simulink model "dvbs2_stream"  (R2024b)
settings: Solver=FixedStepDiscrete  StartTime=0.0  StopTime=18000/Fs  RelTol=1e-3
PreLoadFcn:
  | Rs = 125e3;
  | Fs = 8*Rs;
  | nsamp = 4096;
  | t = (0:nsamp)/Fs;
  | y = randi(2^8-1,1,2048);
  | ly = length(y);
InitFcn:
  | Rs = 125e3;
  | Fs = 8*Rs;
  | nsamp = 4096;
  | t = (0:nsamp)/Fs;
  | y = randi(2^8-1,1,2048);
  | ly = length(y);
libraries: hdlsllib x132, simulink x41, dspsigops x7, commseqgen3 x5, whdlutilities x5, commhdlcrc x2, dsphdlfiltering2 x1, whdlmod x1, sdrzblksprivate x1
(part 4 of 6)

== system dvbs2_stream/HDL_DUT/Tx/DVB-S2 Tx/PL Frame Generator/RAM FIFO/PL Header FIFO ==
  dataIn : Inport
  validIn : Inport  Port=2
  nextFrameReady : Inport  Port=3
  90x : MATLAB Function  TreatAsAtomicUnit=on
  Delay{1..3,9} (4 alike) : Delay  DelayLength=1
  HDL Counter2 : hdlsllib/Sources/HDL Counter  CountType=Count limited  CountInit=0  CountStep=1  CountMax=2^9 - 1  CountFromType=Initial value  CountFrom=0  CountResetPort=off  CountLoadPort=off  CountEnbPort=on  CountDirPort=off  CountHitOutputPort=off  CountDataType=Unsigned  CountWordLen=nextpow2(450)  CountFracLen=0  CountSampTime=1
  HDL Counter3 : hdlsllib/Sources/HDL Counter  CountType=Count limited  CountInit=0  CountStep=1  CountMax=2^9 - 1  CountFromType=Initial value  CountFrom=0  CountResetPort=off  CountLoadPort=off  CountEnbPort=on  CountDirPort=off  CountHitOutputPort=off  CountDataType=Unsigned  CountWordLen=nextpow2(450)  CountFracLen=0  CountSampTime=1
  No HDL : Subsystem
  Simple Dual Port RAM : hdlsllib/HDL RAMs/Simple Dual Port RAM  ram_size=nextpow2(450)
  dataOut : Outport
  startOut : Outport  Port=2
  endOut : Outport  Port=3
  validOut : Outport  Port=4
  endOut1 : Outport  Port=5
  wires:
  90x/4(endOutm1) -> Delay3/1
  Delay3/1 -> endOut1/1
  Delay2/1 -> endOut/1
  Delay1/1 -> startOut/1
  Delay9/1 -> validOut/1
  Simple Dual Port RAM/1 -> dataOut/1
  nextFrameReady/1 -> 90x/1(trigger)
  90x/3(endOut) -> Delay2/1
  90x/2(startOut) -> Delay1/1
  90x/1(validOut) -> Delay9/1, No HDL/2(rd), HDL Counter3/1
  HDL Counter2/1 -> Simple Dual Port RAM/2
  dataIn/1 -> Simple Dual Port RAM/1
  HDL Counter3/1 -> Simple Dual Port RAM/4
  validIn/1 -> No HDL/1(wr), HDL Counter2/1, Simple Dual Port RAM/3

== system dvbs2_stream/HDL_DUT/Tx/DVB-S2 Tx/PL Frame Generator/RAM FIFO/Pilot Generator ==
  trigger : Inport
  Pilot Block Length Valid Generator : MATLAB Function  TreatAsAtomicUnit=on
  Pilot or Unmodulated Carrier : Constant  Value=fi(exp(1i*pi/4),1,18,16)  SampleTime=1/Rsym
  dataOut : Outport
  endOut : Outport  Port=2
  validOut : Outport  Port=3
  endOut1 : Outport  Port=4
  wires:
  Pilot Block Length Valid Generator/2(endOutm1) -> endOut1/1
  Pilot Block Length Valid Generator/3(validOut) -> validOut/1
  Pilot Block Length Valid Generator/1(endOut) -> endOut/1
  Pilot or Unmodulated Carrier/1 -> dataOut/1
  trigger/1 -> Pilot Block Length Valid Generator/1(trigger)

== system dvbs2_stream/HDL_DUT/Tx/DVB-S2 Tx/BB Frame Generator/BB Header and Data CRC Generator/Data Field Generator/Continuous Streams ==
  dataIn : Inport
  validIn : Inport  Port=2
  frameEnd : Inport  Port=3
  frameStart : Inport  Port=4
  Delay{,1..3} (4 alike) : Delay  DelayLength=8+1+10
  dataOut : Outport
  validOut : Outport  Port=2
  frameEndOut : Outport  Port=3
  frameStartOut : Outport  Port=4
  wires:
  validIn/1 -> Delay1/1
  frameEnd/1 -> Delay2/1
  Delay2/1 -> frameEndOut/1
  Delay3/1 -> frameStartOut/1
  frameStart/1 -> Delay3/1
  Delay1/1 -> validOut/1
  dataIn/1 -> Delay/1
  Delay/1 -> dataOut/1

== system dvbs2_stream/HDL_DUT/Tx/DVB-S2 Tx/BB Frame Generator/BB Header and Data CRC Generator/Data Field Generator/Packetized Streams ==
  dataIn : Inport
  startIn : Inport  Port=2
  endIn : Inport  Port=3
  validIn : Inport  Port=4
  frameEnd : Inport  Port=5
  frameStart : Inport  Port=6
  Delay : Delay  DelayLength=1
  Delay1 : Delay  DelayLength=1
  Delay2 : Delay  DelayLength=8
  Delay3 : Delay  DelayLength=10
  Delay4 : Delay  DelayLength=10
  Discard SYNC : MATLAB Function  TreatAsAtomicUnit=on
  MATLAB Function : MATLAB Function  TreatAsAtomicUnit=on
  Terminator : Terminator
  Terminator1 : Terminator
  User Packet CRC Generator : commhdlcrc/General CRC Generator HDL Optimized  Polynomial=[1 1 1 0 1 0 1 0 1]  InitialState=0  DirectMethod=off  ReflectInput=off  ReflectCRCChecksum=off  FinalXORValue=0  SimulateUsing=Code generation
  pktBits : Outport
  pktValid : Outport  Port=2
  frameEndOut : Outport  Port=3
  frameStartOut : Outport  Port=4
  wires:
  Delay4/1 -> MATLAB Function/2(frameEndIn)
  User Packet CRC Generator/4 -> pktValid/1
  Delay3/1 -> frameStartOut/1
  endIn/1 -> Discard SYNC/3(endIn)
  startIn/1 -> Discard SYNC/2(startIn)
  frameEnd/1 -> Delay/1
  frameStart/1 -> Delay2/1
  User Packet CRC Generator/1 -> pktBits/1
  Delay1/1 -> Delay3/1
  Discard SYNC/2(startOut) -> User Packet CRC Generator/2
  Discard SYNC/3(endOut) -> User Packet CRC Generator/3
  User Packet CRC Generator/2 -> Terminator/1
  User Packet CRC Generator/3 -> MATLAB Function/1(pktEndIn), Terminator1/1
  Discard SYNC/4(validOut) -> User Packet CRC Generator/4
  dataIn/1 -> Discard SYNC/1(dataIn)
  validIn/1 -> Discard SYNC/4(validIn)
  Delay/1 -> Delay4/1
  Delay2/1 -> Delay1/1
  MATLAB Function/1(frameEndOut) -> frameEndOut/1
  Discard SYNC/1(dataOut) -> User Packet CRC Generator/1

== system dvbs2_stream/HDL_DUT/Tx/DVB-S2 Tx/BB Frame Generator/BB Header and Data CRC Generator/No HDL/No HDL ==
  rdy : Inport
  vld : Inport  Port=2
  Assertion : Assertion
  Logical Operator : Logic  AllPortsSameDT=off  OutDataTypeStr=boolean
  Logical Operator1 : Logic  Operator=NOT  AllPortsSameDT=off  OutDataTypeStr=boolean
  Logical Operator2 : Logic  Operator=NOT  AllPortsSameDT=off  OutDataTypeStr=boolean
  wires:
  Logical Operator2/1 -> Assertion/1
  rdy/1 -> Logical Operator1/1
  Logical Operator/1 -> Logical Operator2/1
  vld/1 -> Logical Operator/2
  Logical Operator1/1 -> Logical Operator/1

== system dvbs2_stream/HDL_DUT/Tx/DVB-S2 Tx/BB Frame Generator/Data Store FIFO/No HDL/No HDL ==
  wr : Inport
  full : Inport  Port=2
  ncount : Inport  Port=3
  empty : Inport  Port=4
  rd : Inport  Port=5
  Assertion : Assertion  AssertionFailFcn=warning('push on to a full RAM');  StopWhenAssertionFail=off
  Assertion1 : Assertion  AssertionFailFcn=warning('pop from an empty RAM');  StopWhenAssertionFail=off
  Assertion2 : Assertion  AssertionFailFcn='count exceeded 80'
  Compare To Constant : simulink/Logic and Bit Operations/Compare To Constant  relop=<=  const=80  OutDataTypeStr=boolean
  Display : Display
  Logical Operator : Logic  Operator=NAND  AllPortsSameDT=off  OutDataTypeStr=boolean
  Logical Operator1 : Logic  Operator=NAND  AllPortsSameDT=off  OutDataTypeStr=boolean
  wires:
  Logical Operator1/1 -> Assertion1/1
  wr/1 -> Logical Operator/1
  full/1 -> Logical Operator/2
  ncount/1 -> Compare To Constant/1, Display/1
  empty/1 -> Logical Operator1/1
  Logical Operator/1 -> Assertion/1
  rd/1 -> Logical Operator1/2
  Compare To Constant/1 -> Assertion2/1

== system dvbs2_stream/HDL_DUT/Tx/DVB-S2 Tx/FEC Encoder/DVB-S2 BCH Encoder/Parity Generation/Store and Retrieve Parity ==
  iwr_data : Inport  Partition=on  PartitionDimension=1  PartitionWidth=1  PartitionOffset=0
  iwr_addr : Inport  Port=2
  iwr_enb : Inport  Port=3  Partition=on  PartitionDimension=1  PartitionWidth=1  PartitionOffset=0
  ird_addr : Inport  Port=4
  For Each : ForEach  DisableCoverage=on
  parity RAM : hdlsllib/HDL RAMs/Simple Dual Port RAM  ram_size=3
  ird_data : Outport  ConcatenationDimension=1
  wires:
  ird_addr/1 -> parity RAM/4
  iwr_data/1 -> parity RAM/1
  iwr_addr/1 -> parity RAM/2
  iwr_enb/1 -> parity RAM/3
  parity RAM/1 -> ird_data/1

== system dvbs2_stream/HDL_DUT/Tx/DVB-S2 Tx/Interleaver/DVB-S2 HDL Interleaver/RAM/Single RAM Using Two RAMs ==
  wr_din : Inport
  wr_addr : Inport  Port=2
  wr_en : Inport  Port=3
  rd_addr : Inport  Port=4
  Delay : Delay  DelayLength=1
  Extract Bits : simulink/Logic and Bit Operations/Extract Bits  bitsToExtract=Range of bits  numBits=8  bitIdxRange=[0 15]  outScalingMode=Treat bit field as an integer
  Extract Bits1 : simulink/Logic and Bit Operations/Extract Bits  bitsToExtract=Range of bits  numBits=8  bitIdxRange=16  outScalingMode=Treat bit field as an integer
  Extract Bits2 : simulink/Logic and Bit Operations/Extract Bits  bitsToExtract=Range of bits  numBits=8  bitIdxRange=[0 15]  outScalingMode=Treat bit field as an integer
  Extract Bits3 : simulink/Logic and Bit Operations/Extract Bits  bitsToExtract=Range of bits  numBits=8  bitIdxRange=16  outScalingMode=Treat bit field as an integer
  Logical Operator1 : Logic  Operator=NOT  AllPortsSameDT=off  OutDataTypeStr=boolean
  Logical Operator2 : Logic  AllPortsSameDT=off  OutDataTypeStr=boolean
  Logical Operator3 : Logic  AllPortsSameDT=off  OutDataTypeStr=boolean
  Multiport Switch : MultiPortSwitch  DataPortOrder=Zero-based contiguous  Inputs=2  zeroidx=on  SaturateOnIntegerOverflow=off  InputSameDT=off
  Simple Dual Port RAM : hdlsllib/HDL RAMs/Simple Dual Port RAM  ram_size=nextpow2(ConfigRx.RAMCapacity/2)
  Simple Dual Port RAM1 : hdlsllib/HDL RAMs/Simple Dual Port RAM  ram_size=nextpow2(ConfigRx.RAMCapacity/2)
  rd_dout : Outport
  wires:
  Delay/1 -> Multiport Switch/1
  Multiport Switch/1 -> rd_dout/1
  Simple Dual Port RAM1/1 -> Multiport Switch/3
  Extract Bits3/1 -> Delay/1
  Extract Bits2/1 -> Simple Dual Port RAM1/4, Simple Dual Port RAM/4
  Logical Operator2/1 -> Simple Dual Port RAM1/3
  Logical Operator3/1 -> Simple Dual Port RAM/3
  Logical Operator1/1 -> Logical Operator3/1
  Extract Bits1/1 -> Logical Operator2/1, Logical Operator1/1
  Extract Bits/1 -> Simple Dual Port RAM1/2, Simple Dual Port RAM/2
  Simple Dual Port RAM/1 -> Multiport Switch/2
  wr_din/1 -> Simple Dual Port RAM/1, Simple Dual Port RAM1/1
  rd_addr/1 -> Extract Bits3/1, Extract Bits2/1
  wr_en/1 -> Logical Operator2/2, Logical Operator3/2
  wr_addr/1 -> Extract Bits1/1, Extract Bits/1

== system dvbs2_stream/HDL_DUT/Tx/DVB-S2 Tx/Interleaver/DVB-S2 HDL Interleaver/RAM/Wrap Address ==
  u : Inport
  Add : Sum  Inputs=+-  OutDataTypeStr=Inherit: Same as first input
  Compare To Constant : simulink/Logic and Bit Operations/Compare To Constant  relop=>=  const=ConfigRx.RAMCapacity  OutDataTypeStr=boolean
  Constant : Constant  Value=ConfigRx.RAMCapacity  OutDataTypeStr=Inherit: Inherit via back propagation  SampleTime=Tsamp
  Constant1 : Constant  Value=0  OutDataTypeStr=Inherit: Inherit via back propagation  SampleTime=Tsamp
  Data Type Duplicate : DataTypeDuplicate
  Data Type Duplicate1 : DataTypeDuplicate
  Data Type Conversion : DataTypeConversion  OutDataTypeStr=fixdt(0,nextpow2(ConfigRx.RAMCapacity),0)  SaturateOnIntegerOverflow=off  RndMeth=Floor
  Switch : Switch  Criteria=u2 ~= 0  SaturateOnIntegerOverflow=off  InputSameDT=off
  Switch1 : Switch  Criteria=u2 ~= 0  SaturateOnIntegerOverflow=off  InputSameDT=off
  y : Outport
  wires:
  u/1 -> Switch/3, Data Type Duplicate/1, Add/1, Compare To Constant/1
  Switch/1 -> Data Type Conversion/1
  Compare To Constant/1 -> Switch1/2, Switch/2
  Add/1 -> Switch/1
  Constant/1 -> Switch1/1, Data Type Duplicate1/1, Data Type Duplicate/2
  Data Type Conversion/1 -> y/1
  Switch1/1 -> Add/2
  Constant1/1 -> Data Type Duplicate1/2, Switch1/3

== system dvbs2_stream/HDL_DUT/Tx/DVB-S2 Tx/Interleaver/DVB-S2 HDL Interleaver/RAM Address Generator/Generate and Add Read Base Address ==
  readAddrIn : Inport
  readValidIn : Inport  Port=2
  startIn : Inport  Port=3
  endIn : Inport  Port=4
  Add : Sum  Inputs=|++
  Delay{,1,3..4,18} (5 alike) : Delay  DelayLength=1
  Delay{5..9,11,13..16,19..20} (12 alike) : Delay
  Gain : Gain  Gain=ConfigRx.ShortFrameLen  ParamDataTypeStr=fixdt(0,nextpow2(16200),0)
  HDL Counter : hdlsllib/Sources/HDL Counter  CountType=Count limited  CountInit=0  CountStep=1  CountMax=(ConfigRx.RAMCapacity/ConfigRx.ShortFrameLen) - 1  CountFromType=Initial value  CountFrom=0  CountResetPort=off  CountLoadPort=off  CountEnbPort=on  CountDirPort=off  CountHitOutputPort=off  CountDataType=Unsigned  CountWordLen=nextpow2((ConfigRx.RAMCapacity/ConfigRx.ShortFrameLen) - 1)  CountFracLen=0  CountSampTime=1
  Indicate End of Every ShortFrame Length Samples : Subsystem
  Logical Operator : Logic  AllPortsSameDT=off  OutDataTypeStr=boolean
  No HDL Read Address Debug Scope : Subsystem
      settings: PortSchema="{\"entries\":[{\"content\":{\"sides\":[{\"content\":{\"connectorIds\":[]},\"type\":\"ConnectorPlacement.EquallySpacedRectSide\",\"uuid\":\"46203939-3922-41f1-8ac4-248045cc482a\"},{\"content\":{\"connectorIds\":[],\"side\":\"RIGHT\"},\"type\":\"ConnectorPlacement.EquallySpacedRectSide\",\"uuid\":\"e2b32fd8-ba43-4add-9433-a5e10ef1a6cd\"},{\"content\":{\"connectorIds\":[],\"side\":\"TOP\"},\"type\":\"ConnectorPlacement.EquallySpacedRectSide\",\"uuid\":\"bfa555b4-8f13-4832-b51a-da5c9f2f7d4d\"},{\"content\":{\"connectorIds\":[\"In1\",\"In2\",\"In3\",\"In4\"],\"side\":\"BOTTOM\"},\"type\":\"ConnectorPlacement.EquallySpacedRectSide\",\"uuid\":\"1df13975-2c0e-47d4-aefc-7a99adf3a0bb\"}]},\"type\":\"ConnectorPlacement.EquallySpacedConnector\",\"uuid\":\"18a89938-2c8d-49b5-957c-22a1a70f8f87\"}],\"packageUris\":[\"http://schema.mathworks.com/mf0/Connector/R2020b\"],\"version\":\"1.0\"}"
  Unit Delay Enabled Synchronous3 : hdlsllib/Discrete/Unit Delay Enabled Synchronous  InitialCondition=0.0  SampleTime=-1
  readAddrOut : Outport
  readValidOut : Outport  Port=2
  readStartOut : Outport  Port=3
  readEndOut : Outport  Port=4
  wires:
  Gain/1 -> Delay6/1
  Indicate End of Every ShortFrame Length Samples/1(endIndicate) -> Logical Operator/1
  readAddrIn/1 -> Indicate End of Every ShortFrame Length Samples/1(readAddr), Delay3/1
  HDL Counter/1 -> Delay5/1, No HDL Read Address Debug Scope/1(baseAddrIdx)
  Logical Operator/1 -> HDL Counter/1
  Unit Delay Enabled Synchronous3/1 -> Add/2
  Add/1 -> readAddrOut/1, No HDL Read Address Debug Scope/4(basePlusOffsetAddr)
  readValidIn/1 -> Logical Operator/2, Delay4/1
  endIn/1 -> Delay1/1, Delay/1
  Delay/1 -> Delay7/1
  Delay1/1 -> Delay9/1
  Delay3/1 -> Delay13/1
  Delay4/1 -> Delay14/1
  Delay5/1 -> Gain/1
  Delay6/1 -> Unit Delay Enabled Synchronous3/1
  Delay7/1 -> Delay8/1, No HDL Read Address Debug Scope/2(captureBaseAddrIdx)
  Delay8/1 -> Unit Delay Enabled Synchronous3/2
  Delay9/1 -> Delay11/1
  Delay11/1 -> readEndOut/1
  Delay13/1 -> Delay15/1
  Delay14/1 -> Delay16/1
  Delay15/1 -> Add/1, No HDL Read Address Debug Scope/3(offsetAddr)
  Delay16/1 -> readValidOut/1
  startIn/1 -> Delay18/1
  Delay18/1 -> Delay19/1
  Delay19/1 -> Delay20/1
  Delay20/1 -> readStartOut/1

== system dvbs2_stream/HDL_DUT/Tx/DVB-S2 Tx/Interleaver/DVB-S2 HDL Interleaver/RAM Address Generator/Parameter Store FIFO ==
  writeVal : Inport
  modIdxOut : Inport  Port=2
  codIdxOut : Inport  Port=3
  fecFrameOut : Inport  Port=4
  readVal : Inport  Port=5
  Delay1 : Delay  DelayLength=3
  Delay{6,8..14,21..23,25} (12 alike) : Delay  DelayLength=1
  Delay{3..5,7,15..20,24,26,28..29} (14 alike) : Delay
  Delay2 : Delay  DelayLength=3
  Delay27 : Delay  DelayLength=5
  Fec Frame FIFO : hdlsllib/HDL RAMs/Simple Dual Port RAM  ram_size=log2(8)
  ReadVal Address : hdlsllib/Sources/HDL Counter  CountType=Count limited  CountInit=0  CountStep=1  CountMax=7  CountFromType=Initial value  CountFrom=0  CountResetPort=off  CountLoadPort=off  CountEnbPort=on  CountDirPort=off  CountHitOutputPort=off  CountDataType=Unsigned  CountWordLen=3  CountFracLen=0  CountSampTime=1
  Simple Dual Port RAM2 : hdlsllib/HDL RAMs/Simple Dual Port RAM  ram_size=log2(8)
  WriteVal Address : hdlsllib/Sources/HDL Counter  CountType=Count limited  CountInit=0  CountStep=1  CountMax=7  CountFromType=Initial value  CountFrom=0  CountResetPort=off  CountLoadPort=off  CountEnbPort=on  CountDirPort=off  CountHitOutputPort=off  CountDataType=Unsigned  CountWordLen=3  CountFracLen=0  CountSampTime=1
  cod Idx FIFO : hdlsllib/HDL RAMs/Simple Dual Port RAM  ram_size=log2(8)
  codIdx : Outport
  fecframe : Outport  Port=2
  modIdx : Outport  Port=3
  wires:
  Delay29/1 -> Simple Dual Port RAM2/4
  Delay28/1 -> Simple Dual Port RAM2/3
  Delay26/1 -> Simple Dual Port RAM2/2
  Delay24/1 -> Simple Dual Port RAM2/1
  Delay25/1 -> Delay29/1
  Delay23/1 -> Delay28/1
  Delay21/1 -> Delay26/1
  Delay22/1 -> Delay24/1
  Delay27/1 -> modIdx/1
  ReadVal Address/1 -> Delay10/1, Delay14/1, Delay25/1
  writeVal/1 -> Delay13/1, Delay23/1, WriteVal Address/1, Delay9/1
  WriteVal Address/1 -> Delay8/1, Delay12/1, Delay21/1
  modIdxOut/1 -> Delay22/1
  Simple Dual Port RAM2/1 -> Delay27/1
  readVal/1 -> ReadVal Address/1
  codIdxOut/1 -> Delay6/1
  cod Idx FIFO/1 -> Delay3/1
  fecFrameOut/1 -> Delay11/1
  Fec Frame FIFO/1 -> Delay4/1
  Delay1/1 -> codIdx/1
  Delay2/1 -> fecframe/1
  Delay3/1 -> Delay1/1
  Delay4/1 -> Delay2/1
  Delay5/1 -> cod Idx FIFO/1
  Delay7/1 -> cod Idx FIFO/2
  Delay6/1 -> Delay5/1
  Delay8/1 -> Delay7/1
  Delay9/1 -> Delay15/1
  Delay10/1 -> Delay16/1
  Delay11/1 -> Delay17/1
  Delay12/1 -> Delay18/1
  Delay13/1 -> Delay19/1
  Delay14/1 -> Delay20/1
  Delay15/1 -> cod Idx FIFO/3
  Delay16/1 -> cod Idx FIFO/4
  Delay17/1 -> Fec Frame FIFO/1
  Delay18/1 -> Fec Frame FIFO/2
  Delay19/1 -> Fec Frame FIFO/3
  Delay20/1 -> Fec Frame FIFO/4

== system dvbs2_stream/HDL_DUT/Tx/DVB-S2 Tx/Interleaver/DVB-S2 HDL Interleaver/RAM Address Generator/Read Offset Address ==
  maxR : Inport
  maxC : Inport  Port=2
  modcodIs12 : Inport  Port=3
  wrAddr : Inport  Port=4
  wrEnb : Inport  Port=5
  modIdx : Inport  Port=6
  Compute Read Offset Address : Subsystem
  Delay{,1..7,9} (9 alike) : Delay  DelayLength=4
  Generate Signal for End of Frame : Subsystem
  Read Offset Address Signals Generator : Subsystem
  readAddr : Outport
  readValid : Outport  Port=2
  startOut : Outport  Port=3
  endOut : Outport  Port=4
  wires:
  Delay3/1 -> Read Offset Address Signals Generator/5(wrAddr)
  modIdx/1 -> Delay7/1
  Delay7/1 -> Read Offset Address Signals Generator/7(modIdx)
  modcodIs12/1 -> Delay2/1
  wrAddr/1 -> Delay3/1
  wrEnb/1 -> Delay4/1
  Read Offset Address Signals Generator/6(readValid) -> Delay9/1
  Read Offset Address Signals Generator/4(startOut) -> Delay6/1
  Read Offset Address Signals Generator/5(endOut) -> Delay5/1
  maxC/1 -> Generate Signal for End of Frame/2(maxC), Delay1/1
  maxR/1 -> Generate Signal for End of Frame/1(maxR), Delay/1
  Generate Signal for End of Frame/1(chkwrAddrEnd) -> Read Offset Address Signals Generator/2(chkwrAddrEnd)
  Delay/1 -> Read Offset Address Signals Generator/1(maxR)
  Delay1/1 -> Read Offset Address Signals Generator/3(maxC)
  Delay2/1 -> Read Offset Address Signals Generator/4(modcodIs12)
  Delay4/1 -> Read Offset Address Signals Generator/6(wrEnb)
  Delay5/1 -> endOut/1
  Delay9/1 -> readValid/1
  Compute Read Offset Address/1(addr) -> readAddr/1
  Read Offset Address Signals Generator/1(curCorROut) -> Compute Read Offset Address/1(curR)
  Read Offset Address Signals Generator/2(maxRorCOut) -> Compute Read Offset Address/2(maxC)
  Read Offset Address Signals Generator/3(curRorCOut) -> Compute Read Offset Address/3(curC)
  Delay6/1 -> startOut/1

== system dvbs2_stream/HDL_DUT/Tx/DVB-S2 Tx/Interleaver/DVB-S2 HDL Interleaver/RAM Address Generator/Write Offset Address ==
  fecframe : Inport
  enb : Inport  Port=2
  Compare To Constant : simulink/Logic and Bit Operations/Compare To Constant  relop===  const=ConfigRx.ShortFrameLen - 1  OutDataTypeStr=boolean
  Data Type Duplicate : DataTypeDuplicate
  Data Type Conversion : DataTypeConversion  SaturateOnIntegerOverflow=off  RndMeth=Floor
  Delay{1..12} (12 alike) : Delay  DelayLength=1
  Logical Operator : Logic  Inputs=3  AllPortsSameDT=off  OutDataTypeStr=boolean
  Switch : Switch  Criteria=u2 ~= 0  SaturateOnIntegerOverflow=off  InputSameDT=off
  Write Offset Address Normal Frame : hdlsllib/Sources/HDL Counter  CountType=Count limited  CountInit=0  CountStep=1  CountMax=ConfigRx.NormalFrameLen - 1  CountFromType=Initial value  CountFrom=0  CountResetPort=on  CountLoadPort=off  CountEnbPort=on  CountDirPort=off  CountHitOutputPort=off  CountDataType=Unsigned  CountWordLen=nextpow2(ConfigRx.NormalFrameLen - 1)  CountFracLen=0  CountSampTime=1
  Write Offset Address Short Frame : hdlsllib/Sources/HDL Counter  CountType=Count limited  CountInit=0  CountStep=1  CountMax=ConfigRx.ShortFrameLen - 1  CountFromType=Initial value  CountFrom=0  CountResetPort=off  CountLoadPort=off  CountEnbPort=on  CountDirPort=off  CountHitOutputPort=off  CountDataType=Unsigned  CountWordLen=nextpow2(ConfigRx.ShortFrameLen - 1)  CountFracLen=0  CountSampTime=1
  addr : Outport
  wires:
  enb/1 -> Delay10/1
  Write Offset Address Normal Frame/1 -> Delay2/1, Data Type Duplicate/2
  Write Offset Address Short Frame/1 -> Delay8/1
  Compare To Constant/1 -> Logical Operator/2
  Switch/1 -> addr/1
  Logical Operator/1 -> Delay6/1
  Delay11/1 -> Logical Operator/1, Delay4/1
  Data Type Conversion/1 -> Delay5/1, Data Type Duplicate/1
  Delay5/1 -> Switch/1
  Delay1/1 -> Switch/2
  Delay2/1 -> Switch/3
  Delay3/1 -> Data Type Conversion/1
  Delay4/1 -> Delay1/1
  Delay6/1 -> Write Offset Address Normal Frame/1
  Delay7/1 -> Write Offset Address Normal Frame/2
  Delay8/1 -> Delay3/1, Compare To Constant/1
  Delay9/1 -> Delay7/1, Logical Operator/3
  Delay10/1 -> Write Offset Address Short Frame/1, Delay9/1
  fecframe/1 -> Delay12/1
  Delay12/1 -> Delay11/1

== system dvbs2_stream/HDL_DUT/Tx/DVB-S2 Tx/Interleaver/DVB-S2 HDL Interleaver/RAM Address Generator/nRows and nColumns ==
  captureIn : Inport
  modIdx : Inport  Port=2
  codIdx : Inport  Port=3
  fecFrame : Inport  Port=4
  Compare To Constant : simulink/Logic and Bit Operations/Compare To Constant  relop===  const=1  OutDataTypeStr=boolean
  Compare To Constant1 : simulink/Logic and Bit Operations/Compare To Constant  relop===  const=4  OutDataTypeStr=boolean
  Data Type Duplicate : DataTypeDuplicate
  Data Type Conversion : DataTypeConversion  SaturateOnIntegerOverflow=off  RndMeth=Floor
  Delay{1..14} (14 alike) : Delay
  Logical Operator : Logic  AllPortsSameDT=off  OutDataTypeStr=boolean
  MaxC LUT : Lookup_n-D  NumberOfTableDimensions=1  BreakpointsSpecification=Even spacing  BreakpointsForDimension1=[-5:5]  BreakpointsForDimension1FirstPoint=0  Table=[1 3 4 5]  TableDataTypeStr=fixdt(0,3,0)  InterpMethod=Flat  InternalRulePriority=Speed  OutDataTypeStr=fixdt(0,3,0)  RndMeth=Simplest
  MaxR Normal LUT : Lookup_n-D  NumberOfTableDimensions=1  BreakpointsSpecification=Even spacing  BreakpointsForDimension1=[-5:5]  BreakpointsForDimension1FirstPoint=0  Table=64800./[1 3 4 5]  TableDataTypeStr=fixdt(0,nextpow2(64800),0)  InterpMethod=Flat  InternalRulePriority=Speed  OutDataTypeStr=fixdt(0,nextpow2(64800),0)  RndMeth=Simplest
  MaxR Short LUT : Lookup_n-D  NumberOfTableDimensions=1  BreakpointsSpecification=Even spacing  BreakpointsForDimension1=[-5:5]  BreakpointsForDimension1FirstPoint=0  Table=16200./[1 3 4 5]  TableDataTypeStr=fixdt(0,nextpow2(16200),0)  InterpMethod=Flat  InternalRulePriority=Speed  OutDataTypeStr=fixdt(0,nextpow2(16200),0)  RndMeth=Simplest
  maxR_switch : MultiPortSwitch  DataPortOrder=Zero-based contiguous  Inputs=2  zeroidx=on  SaturateOnIntegerOverflow=off  InputSameDT=off
  captureOut : Outport
  modIdxOut : Outport  Port=2
  codIdxOut : Outport  Port=3
  fecFrameOut : Outport  Port=4
  maxR : Outport  Port=5
  maxC : Outport  Port=6
  isMODOCD12 : Outport  Port=7
  wires:
  MaxR Normal LUT/1 -> Delay14/1
  Data Type Conversion/1 -> Data Type Duplicate/2, maxR_switch/3
  MaxR Short LUT/1 -> Delay13/1
  fecFrame/1 -> Delay1/1
  MaxC LUT/1 -> Delay12/1
  maxR_switch/1 -> maxR/1
  modIdx/1 -> Delay5/1, Delay11/1, Delay10/1, Delay9/1
  Compare To Constant1/1 -> Logical Operator/2
  Logical Operator/1 -> isMODOCD12/1
  codIdx/1 -> Delay6/1
  Compare To Constant/1 -> Logical Operator/1
  captureIn/1 -> Delay2/1
  Delay1/1 -> Delay3/1
  Delay2/1 -> Delay4/1
  Delay3/1 -> fecFrameOut/1, maxR_switch/1
  Delay4/1 -> captureOut/1
  Delay5/1 -> Delay7/1
  Delay6/1 -> Delay8/1
  Delay7/1 -> modIdxOut/1, Compare To Constant/1
  Delay8/1 -> codIdxOut/1, Compare To Constant1/1
  Delay9/1 -> MaxR Normal LUT/1
  Delay10/1 -> MaxR Short LUT/1
  Delay11/1 -> MaxC LUT/1
  Delay12/1 -> maxC/1
  Delay13/1 -> Data Type Conversion/1
  Delay14/1 -> Data Type Duplicate/1, maxR_switch/2

== system dvbs2_stream/HDL_DUT/Tx/DVB-S2 Tx/PL Frame Generator/PL Data Scrambler/PL Scrambler Gold Sequence Generator/Subsystem ==
  note: The initial output of these outports are set to 0 as this is an enabled subsystem
  reset : Inport
  Enable : EnablePort
  X PN Generator M_n : commseqgen3/PN Sequence Generator  poly='z^18+z^7+1'  ini_sta=[zeros(1,17) 1]  outBitMaskSource=Dialog parameter  shift=n  outVarSiz=off  maxOutSizeMode=Dialog parameter  maxOutSize=[10 1]  Ts=-1  sampPerFrame=1  reset=on  bitPackedOutputs=off  outDataType=boolean  numPackedBits=8  bitPackDataSigned=off  bitPackedOutDType=double
  X PN Generator M_nplus131072 : commseqgen3/PN Sequence Generator  poly='z^18+z^7+1'  ini_sta=[zeros(1,17) 1]  outBitMaskSource=Dialog parameter  shift=n+131072  outVarSiz=off  maxOutSizeMode=Dialog parameter  maxOutSize=[10 1]  Ts=-1  sampPerFrame=1  reset=on  bitPackedOutputs=off  outDataType=boolean  numPackedBits=8  bitPackDataSigned=off  bitPackedOutDType=double
  Y PN Generator M_0 : commseqgen3/PN Sequence Generator  poly='z^18 + z^10 + z^7 + z^5 + 1'  ini_sta=ones(1,18)  outBitMaskSource=Dialog parameter  shift=0  outVarSiz=off  maxOutSizeMode=Dialog parameter  maxOutSize=[10 1]  Ts=-1  sampPerFrame=1  reset=on  bitPackedOutputs=off  outDataType=boolean  numPackedBits=8  bitPackDataSigned=off  bitPackedOutDType=double
  Y PN Generator M_131072 : commseqgen3/PN Sequence Generator  poly='z^18 + z^10 + z^7 + z^5 + 1'  ini_sta=ones(1,18)  outBitMaskSource=Dialog parameter  shift=131072  outVarSiz=off  maxOutSizeMode=Dialog parameter  maxOutSize=[10 1]  Ts=-1  sampPerFrame=1  reset=on  bitPackedOutputs=off  outDataType=boolean  numPackedBits=8  bitPackDataSigned=off  bitPackedOutDType=double
  xMnp131072 : Outport  InitialOutput=0
  yM131072 : Outport  Port=2  InitialOutput=0
  xMn : Outport  Port=3  InitialOutput=0
  yM0 : Outport  Port=4  InitialOutput=0
  wires:
  X PN Generator M_nplus131072/1 -> xMnp131072/1
  Y PN Generator M_0/1 -> yM0/1
  reset/1 -> X PN Generator M_nplus131072/1, Y PN Generator M_0/1, X PN Generator M_n/1, Y PN Generator M_131072/1
  X PN Generator M_n/1 -> xMn/1
  Y PN Generator M_131072/1 -> yM131072/1

== system dvbs2_stream/HDL_DUT/Tx/DVB-S2 Tx/PL Frame Generator/PL Header Generator/PL Header Bits Generator/PLSC Generator ==
  bit7 : Inport
  bits1to6 : Inport  Port=2
  bitsStart : Inport  Port=3
  bitsValidIn : Inport  Port=4
  Bi Orthogonal Coding (32,6) : Subsystem
  Data Type Conversion : DataTypeConversion  OutDataTypeStr=boolean  SaturateOnIntegerOverflow=off  RndMeth=Floor
  Delay : Delay  DelayLength=5
  Delay1 : Delay  DelayLength=5
  Delay2 : Delay  DelayLength=1
  Delay3 : Delay  DelayLength=1
  Delay4 : Delay  DelayLength=5
  HDL Counter : hdlsllib/Sources/HDL Counter  CountType=Count limited  CountInit=0  CountStep=1  CountMax=1  CountFromType=Initial value  CountFrom=0  CountResetPort=off  CountLoadPort=off  CountEnbPort=on  CountDirPort=off  CountHitOutputPort=off  CountDataType=Unsigned  CountWordLen=1  CountFracLen=0  CountSampTime=1
  Logical Operator : Logic  Operator=XOR  AllPortsSameDT=off  OutDataTypeStr=boolean
  PLSC Scrambler : Subsystem
  Repeat : dspsigops/Repeat  FactorSource=Dialog parameter  N=2  Nmax=16  RateOptions=Allow multirate processing  ic=0  mode=Unused parameter value
  Repeat1 : dspsigops/Repeat  FactorSource=Dialog parameter  N=2  Nmax=16  RateOptions=Allow multirate processing  ic=0  mode=Unused parameter value
  Repeat2 : dspsigops/Repeat  FactorSource=Dialog parameter  N=2  Nmax=16  RateOptions=Allow multirate processing  ic=0  mode=Unused parameter value
  Serialize on trigger : MATLAB Function  TreatAsAtomicUnit=on
  Switch : Switch  Criteria=u2 ~= 0  SaturateOnIntegerOverflow=off  InputSameDT=off
  Terminator : Terminator
  Unit Delay Enabled Synchronous : hdlsllib/Discrete/Unit Delay Enabled Synchronous  InitialCondition=0.0  SampleTime=-1
  Upsample : dspsigops/Upsample  FactorSource=Dialog parameter  N=2  Nmax=16  phase=0  RateOptions=Allow multirate processing  ic=0  mode=Unused parameter value
  bitsOut : Outport
  bitsValid : Outport  Port=2
  endOfPLSC : Outport  Port=3
  wires:
  PLSC Scrambler/4(endOfPLSC) -> endOfPLSC/1
  PLSC Scrambler/3(resetOut) -> Terminator/1
  PLSC Scrambler/2(validOut) -> bitsValid/1
  PLSC Scrambler/1(dataOut) -> bitsOut/1
  Upsample/1 -> PLSC Scrambler/3(resetIn)
  Delay4/1 -> Upsample/1
  Serialize on trigger/3(startOut) -> Delay4/1
  Delay3/1 -> PLSC Scrambler/2(validIn)
  Delay2/1 -> PLSC Scrambler/1(dataIn)
  Delay1/1 -> Repeat1/1
  Delay/1 -> Repeat/1
  bits1to6/1 -> Bi Orthogonal Coding (32,6)/2(bitsIn)
  Switch/1 -> Delay2/1
  Unit Delay Enabled Synchronous/1 -> Repeat2/1
  Bi Orthogonal Coding (32,6)/1(bitsOut) -> Serialize on trigger/1(data)
  Repeat/1 -> Data Type Conversion/1
  Repeat1/1 -> HDL Counter/1, Delay3/1
  bitsValidIn/1 -> Bi Orthogonal Coding (32,6)/3(bitsValidIn)
  Data Type Conversion/1 -> Switch/3, Logical Operator/2
  Serialize on trigger/2(validOut) -> Delay1/1
  bitsStart/1 -> Bi Orthogonal Coding (32,6)/1(bitsStart), Unit Delay Enabled Synchronous/2
  HDL Counter/1 -> Switch/2
  bit7/1 -> Unit Delay Enabled Synchronous/1
  Serialize on trigger/1(dataOut) -> Delay/1
  Logical Operator/1 -> Switch/1
  Bi Orthogonal Coding (32,6)/2(done) -> Serialize on trigger/2(trigger)
  Repeat2/1 -> Logical Operator/1

== system dvbs2_stream/HDL_DUT/Tx/DVB-S2 Tx/PL Frame Generator/PL Header Generator/PL Header Bits Generator/SOF Generator ==
  trigger : Inport
  Compare To Constant : simulink/Logic and Bit Operations/Compare To Constant  relop===  const=0  OutDataTypeStr=boolean
  Data Type Conversion : DataTypeConversion  OutDataTypeStr=boolean  SaturateOnIntegerOverflow=off  RndMeth=Floor
  Logical Operator : Logic  AllPortsSameDT=off  OutDataTypeStr=boolean
  SOF Sequence : Lookup_n-D  NumberOfTableDimensions=1  BreakpointsSpecification=Even spacing  BreakpointsForDimension1=[-5:5]  BreakpointsForDimension1FirstPoint=0  Table=config.SOF  TableDataTypeStr=Inherit: Inherit from 'Table data'  InterpMethod=Flat  DiagnosticForOutOfRangeInput=Warning  InternalRulePriority=Speed  OutDataTypeStr=Inherit: Inherit from 'Table data'  RndMeth=Simplest
  SOF Sequence LUT Address Generator : MATLAB Function  TreatAsAtomicUnit=on
  Upsample : dspsigops/Upsample  FactorSource=Dialog parameter  N=2  Nmax=16  phase=0  RateOptions=Allow multirate processing  ic=0  mode=Unused parameter value
  dataOut : Outport
  validOut : Outport  Port=2
  startOfSOF : Outport  Port=3
  wires:
  Upsample/1 -> SOF Sequence LUT Address Generator/1(trigger)
  trigger/1 -> Upsample/1
  Compare To Constant/1 -> Logical Operator/1
  Logical Operator/1 -> startOfSOF/1
  Data Type Conversion/1 -> dataOut/1
  SOF Sequence LUT Address Generator/2(valid) -> validOut/1, Logical Operator/2
  SOF Sequence/1 -> Data Type Conversion/1
  SOF Sequence LUT Address Generator/1(LUTAddr) -> SOF Sequence/1, Compare To Constant/1

== system dvbs2_stream/HDL_DUT/Tx/DVB-S2 Tx/PL Frame Generator/RAM FIFO/PL Data FIFO/Dummy Frame Generator ==
  frameLength : Inport
  EOF : Inport  Port=2
  readyNxtFrame : Inport  Port=3
  Compare To Constant : simulink/Logic and Bit Operations/Compare To Constant  relop=~=  const=0  OutDataTypeStr=boolean
  Compare To Constant1 : simulink/Logic and Bit Operations/Compare To Constant  relop=<=  const=(64800/5 + 16200/2)/2  OutDataTypeStr=boolean
  Compare To Constant2 : simulink/Logic and Bit Operations/Compare To Constant  relop=<  const=90  OutDataTypeStr=boolean
  Compare To Constant3 : simulink/Logic and Bit Operations/Compare To Constant  relop===  const=0  OutDataTypeStr=boolean
  Compare To Constant4 : simulink/Logic and Bit Operations/Compare To Constant  relop===  const=89  OutDataTypeStr=boolean
  Constant : Constant  Value=fi(exp(1i*pi/4),1,18,16)  SampleTime=1/Rsym
  Data Type Conversion : DataTypeConversion  OutDataTypeStr=fixdt(0,nextpow2(90),0)  SaturateOnIntegerOverflow=off  RndMeth=Floor
  Dummy Frame Header LUT Address Generator : MATLAB Function  TreatAsAtomicUnit=on
  Dummy Frame Normal Header : Lookup_n-D  NumberOfTableDimensions=1  BreakpointsSpecification=Even spacing  BreakpointsForDimension1=[-5:5]  BreakpointsForDimension1FirstPoint=0  Table=config.dummyFramePLHeaderptruefnormal  TableDataTypeStr=fixdt(1,18,16)  InterpMethod=Flat  InternalRulePriority=Speed  OutDataTypeStr=fixdt(1,18,16)  RndMeth=Simplest
      mask init:
      | Simulink.suppressDiagnostic(gcb, 'SimulinkFixedPoint:util:fxpParameterPrecisionLoss');
  Dummy Frame Short Header : Lookup_n-D  NumberOfTableDimensions=1  BreakpointsSpecification=Even spacing  BreakpointsForDimension1=[-5:5]  BreakpointsForDimension1FirstPoint=0  Table=config.dummyFramePLHeaderptruefshort  TableDataTypeStr=fixdt(1,18,16)  InterpMethod=Flat  InternalRulePriority=Speed  OutDataTypeStr=fixdt(1,18,16)  RndMeth=Simplest
      mask init:
      | Simulink.suppressDiagnostic(gcb, 'SimulinkFixedPoint:util:fxpParameterPrecisionLoss');
  Logical Operator : Logic  AllPortsSameDT=off  OutDataTypeStr=boolean
  Logical Operator1 : Logic  AllPortsSameDT=off  OutDataTypeStr=boolean
  Logical Operator2 : Logic  AllPortsSameDT=off  OutDataTypeStr=boolean
  Switch : Switch  Criteria=u2 ~= 0  SaturateOnIntegerOverflow=off  InputSameDT=off
  Switch1 : Switch  Criteria=u2 ~= 0  SaturateOnIntegerOverflow=off  InputSameDT=off
  data : Outport
  valid1 : Outport  Port=2
  valid : Outport  Port=3
  headerStart : Outport  Port=4
  headerEnd : Outport  Port=5
  wires:
  Logical Operator2/1 -> headerEnd/1
  Logical Operator1/1 -> headerStart/1
  Compare To Constant4/1 -> Logical Operator2/2
  Compare To Constant3/1 -> Logical Operator1/2
  Data Type Conversion/1 -> Dummy Frame Normal Header/1, Dummy Frame Short Header/1
  Dummy Frame Header LUT Address Generator/2(validm2) -> valid1/1
  EOF/1 -> Dummy Frame Header LUT Address Generator/2(EOF)
  readyNxtFrame/1 -> Dummy Frame Header LUT Address Generator/1(nextFrameReady)
  Constant/1 -> Switch1/3
  Switch1/1 -> data/1
  Compare To Constant2/1 -> Switch1/2
  Switch/1 -> Switch1/1
  Dummy Frame Header LUT Address Generator/1(countOut) -> Compare To Constant2/1, Compare To Constant3/1, Compare To Constant4/1, Data Type Conversion/1
  Dummy Frame Header LUT Address Generator/3(valid) -> valid/1, Logical Operator1/1, Logical Operator2/1
  Dummy Frame Normal Header/1 -> Switch/3
  Dummy Frame Short Header/1 -> Switch/1
  Logical Operator/1 -> Switch/2
  Compare To Constant1/1 -> Logical Operator/2
  Compare To Constant/1 -> Logical Operator/1
  frameLength/1 -> Compare To Constant/1, Compare To Constant1/1

== system dvbs2_stream/HDL_DUT/Tx/DVB-S2 Tx/PL Frame Generator/RAM FIFO/PL Data FIFO/Frame Length FIFO ==
  dataIn : Inport
  validIn : Inport  Port=2
  pop : Inport  Port=3
  HDL Counter2 : hdlsllib/Sources/HDL Counter  CountType=Count limited  CountInit=0  CountStep=1  CountMax=2^4 - 1  CountFromType=Initial value  CountFrom=0  CountResetPort=off  CountLoadPort=off  CountEnbPort=on  CountDirPort=off  CountHitOutputPort=off  CountDataType=Unsigned  CountWordLen=4  CountFracLen=0  CountSampTime=1
  HDL Counter3 : hdlsllib/Sources/HDL Counter  CountType=Count limited  CountInit=0  CountStep=1  CountMax=2^4 - 1  CountFromType=Initial value  CountFrom=0  CountResetPort=off  CountLoadPort=off  CountEnbPort=on  CountDirPort=off  CountHitOutputPort=off  CountDataType=Unsigned  CountWordLen=4  CountFracLen=0  CountSampTime=1
  No HDL : Subsystem
  Simple Dual Port RAM : hdlsllib/HDL RAMs/Simple Dual Port RAM  ram_size=4
  dataOut : Outport
  wires:
  validIn/1 -> No HDL/1(wr), Simple Dual Port RAM/3, HDL Counter2/1
  HDL Counter3/1 -> Simple Dual Port RAM/4
  dataIn/1 -> Simple Dual Port RAM/1
  HDL Counter2/1 -> Simple Dual Port RAM/2
  pop/1 -> No HDL/2(rd), HDL Counter3/1
  Simple Dual Port RAM/1 -> dataOut/1

== system dvbs2_stream/HDL_DUT/Tx/DVB-S2 Tx/PL Frame Generator/RAM FIFO/PL Data FIFO/No HDL ==
  wr : Inport
  rd : Inport  Port=2
  No HDL : Subsystem
  RAM status : MATLAB Function  TreatAsAtomicUnit=on
  wires:
  rd/1 -> No HDL/5(rd), RAM status/2(rd)
  RAM status/1(full) -> No HDL/2(full)
  RAM status/3(empty) -> No HDL/4(empty)
  wr/1 -> No HDL/1(wr), RAM status/1(wr)
  RAM status/2(ncount) -> No HDL/3(ncount)

== system dvbs2_stream/HDL_DUT/Tx/DVB-S2 Tx/PL Frame Generator/RAM FIFO/PL Header FIFO/No HDL ==
  wr : Inport
  rd : Inport  Port=2
  No HDL : Subsystem
  RAM status : MATLAB Function  TreatAsAtomicUnit=on
  wires:
  RAM status/3(empty) -> No HDL/4(empty)
  rd/1 -> No HDL/5(rd), RAM status/2(rd)
  RAM status/1(full) -> No HDL/2(full)
  wr/1 -> RAM status/1(wr), No HDL/1(wr)
  RAM status/2(ncount) -> No HDL/3(ncount)

== system dvbs2_stream/HDL_DUT/Tx/DVB-S2 Tx/Interleaver/DVB-S2 HDL Interleaver/RAM Address Generator/Generate and Add Read Base Address/Indicate End of Every ShortFrame Length Samples ==
  readAddr : Inport
  Compare To Constant : simulink/Logic and Bit Operations/Compare To Constant  relop===  const=ConfigRx.ShortFrameLen - 1  OutDataTypeStr=boolean
  Compare To Constant1 : simulink/Logic and Bit Operations/Compare To Constant  relop===  const=ConfigRx.ShortFrameLen*2 - 1  OutDataTypeStr=boolean
  Compare To Constant2 : simulink/Logic and Bit Operations/Compare To Constant  relop===  const=ConfigRx.ShortFrameLen*3 - 1  OutDataTypeStr=boolean
  Compare To Constant3 : simulink/Logic and Bit Operations/Compare To Constant  relop===  const=ConfigRx.ShortFrameLen*4 - 1  OutDataTypeStr=boolean
  Logical Operator1 : Logic  Operator=OR  Inputs=4  AllPortsSameDT=off  OutDataTypeStr=boolean
  endIndicate : Outport
  wires:
  readAddr/1 -> Compare To Constant1/1, Compare To Constant/1, Compare To Constant2/1, Compare To Constant3/1
  Compare To Constant2/1 -> Logical Operator1/3
  Compare To Constant1/1 -> Logical Operator1/2
  Compare To Constant3/1 -> Logical Operator1/4
  Compare To Constant/1 -> Logical Operator1/1
  Logical Operator1/1 -> endIndicate/1

== system dvbs2_stream/HDL_DUT/Tx/DVB-S2 Tx/Interleaver/DVB-S2 HDL Interleaver/RAM Address Generator/Generate and Add Read Base Address/No HDL Read Address Debug Scope ==
  note: Connect these line to Time scope to visualize signals
  note: For Deinterleaver :
  note: Offset Address :
      | Each ramp signal in the time scope indicates a column pickup.
      | 1,3,4,5 ramp signals in constant base address index indicates a frame demodulated from QPSK, 8 PSK, 16 APSK, 32 APSK symbols respectively.
      | The height of the ramps indicates a normal or a short frame
  note: This subsystem is a copy of
      | Wrap Address subsystem
      | in the RAM subsystem
  note: Base Address Index:
      | Remains constant till the end of the frame.
      | changes by 1 after every short and by 4 after every normal frame
  baseAddrIdx : Inport
  captureBaseAddrIdx : Inport  Port=2
  offsetAddr : Inport  Port=3
  basePlusOffsetAddr : Inport  Port=4
  Add1 : Sum  Inputs=+-|
  Delay1 : Delay
  Delay14 : Delay  DelayLength=4
  Terminator{,1..4} (5 alike) : Terminator
  Unit Delay Enabled Synchronous : hdlsllib/Discrete/Unit Delay Enabled Synchronous  InitialCondition=0.0  SampleTime=-1
  Wrap Address : Subsystem
  wires:
  baseAddrIdx/1 -> Delay14/1
  Wrap Address/1(y) -> Terminator3/1, Add1/2  "Wrapped Actual Address"
  captureBaseAddrIdx/1 -> Delay1/1
  Add1/1 -> Terminator4/1  "Actual Address - Wrapped Actual Address"
  Unit Delay Enabled Synchronous/1 -> Terminator1/1  "Base Address Index"
  offsetAddr/1 -> Terminator/1  "Offset Address"
  basePlusOffsetAddr/1 -> Wrap Address/1(u), Terminator2/1, Add1/1  "Actual Address = Base Address Index * 16200 + Offset Address"
  Delay14/1 -> Unit Delay Enabled Synchronous/1
  Delay1/1 -> Unit Delay Enabled Synchronous/2

== system dvbs2_stream/HDL_DUT/Tx/DVB-S2 Tx/Interleaver/DVB-S2 HDL Interleaver/RAM Address Generator/Read Offset Address/Compute Read Offset Address ==
  curR : Inport
  maxC : Inport  Port=2
  curC : Inport  Port=3
  Add : Sum  OutDataTypeStr=Inherit: Same as first input
  Delay1 : Delay  DelayLength=1
  Delay2 : Delay
  Delay3 : Delay
  Delay4 : Delay  DelayLength=1
  Delay5 : Delay  DelayLength=1
  Delay8 : Delay
  Product : Product  OutDataTypeStr=fixdt('ufix17')
  addr : Outport
  wires:
  Add/1 -> Delay5/1
  Delay2/1 -> Product/2
  Product/1 -> Delay1/1
  maxC/1 -> Delay2/1
  curR/1 -> Delay8/1
  Delay3/1 -> Delay4/1
  Delay8/1 -> Product/1
  curC/1 -> Delay3/1
  Delay1/1 -> Add/1
  Delay4/1 -> Add/2
  Delay5/1 -> addr/1

== system dvbs2_stream/HDL_DUT/Tx/DVB-S2 Tx/Interleaver/DVB-S2 HDL Interleaver/RAM Address Generator/Read Offset Address/Generate Signal for End of Frame ==
  maxR : Inport
  maxC : Inport  Port=2
  Add : Sum  Inputs=+-  OutDataTypeStr=Inherit: Same as first input
  Compare To Constant : simulink/Logic and Bit Operations/Compare To Constant  relop=~=  const=0  OutDataTypeStr=boolean
  Constant : Constant  OutDataTypeStr=fixdt('ufix1')  SampleTime=Tsamp
  Constant1 : Constant  Value=0  OutDataTypeStr=fixdt('ufix1')  SampleTime=Tsamp
  Delay : Delay
  Delay1 : Delay
  Delay2 : Delay  DelayLength=1
  Delay4 : Delay  DelayLength=1
  Product : Product  OutDataTypeStr=Inherit: Same as first input
  Switch : Switch  Criteria=u2 > Threshold  SaturateOnIntegerOverflow=off  InputSameDT=off
  chkwrAddrEnd : Outport
  wires:
  Product/1 -> Delay2/1
  maxC/1 -> Delay1/1
  Delay4/1 -> chkwrAddrEnd/1
  Delay/1 -> Product/1
  Delay1/1 -> Product/2
  Add/1 -> Delay4/1
  Constant/1 -> Switch/1
  maxR/1 -> Delay/1
  Delay2/1 -> Compare To Constant/1, Add/1
  Switch/1 -> Add/2
  Constant1/1 -> Switch/3
  Compare To Constant/1 -> Switch/2

== system dvbs2_stream/HDL_DUT/Tx/DVB-S2 Tx/Interleaver/DVB-S2 HDL Interleaver/RAM Address Generator/Read Offset Address/Read Offset Address Signals Generator ==
  maxR : Inport
  chkwrAddrEnd : Inport  Port=2
  maxC : Inport  Port=3
  modcodIs12 : Inport  Port=4
  wrAddr : Inport  Port=5
  wrEnb : Inport  Port=6
  modIdx : Inport  Port=7
  Control Logic : MATLAB Function  TreatAsAtomicUnit=on
  FIFO 3 Variables : Subsystem
  Logical Operator : Logic  AllPortsSameDT=off  OutDataTypeStr=boolean
  Relational Operator : RelationalOperator  Operator===  OutDataTypeStr=boolean  RndMeth=Simplest  InputSameDT=off
  Subsystem : Subsystem
      settings: LibrarySourceBlock=|
      | hdlsllib/Ports &
      | Subsystems/Subsystem
  Terminator : Terminator
  Terminator1 : Terminator
  curCorROut : Outport
  maxRorCOut : Outport  Port=2
  curRorCOut : Outport  Port=3
  startOut : Outport  Port=4
  endOut : Outport  Port=5
  readValid : Outport  Port=6
  wires:
  Control Logic/8(cnt8) -> Terminator1/1
  modIdx/1 -> Control Logic/7(modIdx)
  Control Logic/6(endOut) -> endOut/1, FIFO 3 Variables/3(pop)
  wrAddr/1 -> Relational Operator/2, Control Logic/5(wrAddr)
  modcodIs12/1 -> FIFO 3 Variables/5(modcodis12)
  wrEnb/1 -> Logical Operator/2, Control Logic/6(wrEnb)
  maxC/1 -> FIFO 3 Variables/4(maxC)
  maxR/1 -> FIFO 3 Variables/1(maxR)
  Control Logic/1(curCorROut) -> curCorROut/1
  Control Logic/2(maxRorCOut) -> maxRorCOut/1
  Control Logic/3(curRorCOut) -> curRorCOut/1
  Control Logic/4(modcodIs12Out) -> Terminator/1
  Control Logic/5(startOut) -> startOut/1
  Control Logic/7(readValid) -> readValid/1
  chkwrAddrEnd/1 -> Control Logic/2(chkwrAddrEnd), Subsystem/1(chkwrAddrEnd)
  Logical Operator/1 -> FIFO 3 Variables/2(push)
  Relational Operator/1 -> Logical Operator/1
  FIFO 3 Variables/2(vMaxC) -> Control Logic/3(vMaxC)
  FIFO 3 Variables/1(vMaxR) -> Control Logic/1(vMaxR)
  FIFO 3 Variables/3(vMODCODis12) -> Control Logic/4(vModCodIs12)
  Subsystem/1(Out1) -> Relational Operator/1

== system dvbs2_stream/HDL_DUT/Tx/DVB-S2 Tx/PL Frame Generator/PL Header Generator/PL Header Bits Generator/PLSC Generator/Bi Orthogonal Coding (32,6) ==
  bitsStart : Inport
  bitsIn : Inport  Port=2
  bitsValidIn : Inport  Port=3
  1-D Lookup Table : Lookup_n-D  NumberOfTableDimensions=1  BreakpointsSpecification=Even spacing  BreakpointsForDimension1=[-5:5]  BreakpointsForDimension1FirstPoint=0  Table=config.genMatLUT  TableDataTypeStr=Inherit: Inherit from 'Table data'  InterpMethod=Flat  DiagnosticForOutOfRangeInput=Warning  InternalRulePriority=Speed  OutDataTypeStr=Inherit: Inherit from 'Table data'  RndMeth=Simplest
  Bitwise Operator : simulink/Logic and Bit Operations/Bitwise Operator  logicop=XOR  UseBitMask=off  NumInputPorts=2  BitMask=bin2dec('11011001')  BitMaskRealWorld=Stored Integer
  Compare To Constant : simulink/Logic and Bit Operations/Compare To Constant  relop===  const=5  OutDataTypeStr=boolean
  Constant : Constant  Value=0  OutDataTypeStr=uint32  SampleTime=2/(Rsym)
  Delay : Delay  DelayLength=1
  Delay1 : Delay  DelayLength=1
  HDL Counter : hdlsllib/Sources/HDL Counter  CountType=Count limited  CountInit=0  CountStep=1  CountMax=5  CountFromType=Initial value  CountFrom=0  CountResetPort=on  CountLoadPort=off  CountEnbPort=on  CountDirPort=off  CountHitOutputPort=off  CountDataType=Unsigned  CountWordLen=nextpow2(5)  CountFracLen=0  CountSampTime=1
  Integer to Bit Convertor : Subsystem
  Logical Operator : Logic  AllPortsSameDT=off  OutDataTypeStr=boolean
  Signal Specification : SignalSpecification  OutDataTypeStr=uint32
  Switch : Switch  Criteria=u2 ~= 0  SaturateOnIntegerOverflow=off  InputSameDT=off
  Unit Delay Enabled Synchronous : hdlsllib/Discrete/Unit Delay Enabled Synchronous  InitialCondition=0.0  SampleTime=-1
  Unit Delay Enabled Resettable Synchronous : hdlsllib/Discrete/Unit Delay Enabled Resettable Synchronous  InitialCondition=0.0  SampleTime=-1
  bitsOut : Outport
  done : Outport  Port=2
  wires:
  HDL Counter/1 -> 1-D Lookup Table/1, Compare To Constant/1
  1-D Lookup Table/1 -> Switch/1
  bitsValidIn/1 -> Delay/1
  Delay/1 -> HDL Counter/2, Unit Delay Enabled Resettable Synchronous/2, Logical Operator/2
  bitsIn/1 -> Delay1/1
  bitsStart/1 -> HDL Counter/1
  Constant/1 -> Switch/3
  Delay1/1 -> Switch/2
  Switch/1 -> Bitwise Operator/2
  Bitwise Operator/1 -> Unit Delay Enabled Resettable Synchronous/1, Unit Delay Enabled Synchronous/1
  Compare To Constant/1 -> Logical Operator/1
  Signal Specification/1 -> Bitwise Operator/1
  Integer to Bit Convertor/1(dataOut) -> bitsOut/1
  Unit Delay Enabled Resettable Synchronous/1 -> Signal Specification/1
  Unit Delay Enabled Synchronous/1 -> Integer to Bit Convertor/1(dataIn)
  Logical Operator/1 -> Unit Delay Enabled Resettable Synchronous/3, Unit Delay Enabled Synchronous/2, done/1

== system dvbs2_stream/HDL_DUT/Tx/DVB-S2 Tx/PL Frame Generator/PL Header Generator/PL Header Bits Generator/PLSC Generator/PLSC Scrambler ==
  dataIn : Inport
  validIn : Inport  Port=2
  resetIn : Inport  Port=3
  1-D Lookup Table : Lookup_n-D  NumberOfTableDimensions=1  LookupTableObject=''  BreakpointsSpecification=Even spacing  BreakpointsForDimension1=[-5:5]  BreakpointsForDimension1FirstPoint=0  BreakpointsForDimension2FirstPoint=10  BreakpointsForDimension2Spacing=12  IndexSearchMethod=Evenly spaced points  Table=config.PLSCScramLUT  TableDataTypeStr=Inherit: Inherit from 'Table data'  InterpMethod=Flat  DiagnosticForOutOfRangeInput=Error  InternalRulePriority=Speed  OutDataTypeStr=Inherit: Inherit from 'Table data'  RndMeth=Simplest
  Compare To Constant : simulink/Logic and Bit Operations/Compare To Constant  relop===  const=63  OutDataTypeStr=boolean
  Data Type Conversion : DataTypeConversion  OutDataTypeStr=boolean  SaturateOnIntegerOverflow=off  RndMeth=Floor
  Logical Operator : Logic  Operator=XOR  AllPortsSameDT=off  OutDataTypeStr=boolean
  Logical Operator1 : Logic  AllPortsSameDT=off  OutDataTypeStr=boolean
  PLSC Valid Counter : hdlsllib/Sources/HDL Counter  CountType=Count limited  CountInit=0  CountStep=1  CountMax=length(config.PLSCScramLUT)-1  CountFromType=Initial value  CountFrom=0  CountResetPort=on  CountLoadPort=off  CountEnbPort=on  CountDirPort=off  CountHitOutputPort=off  CountDataType=Unsigned  CountWordLen=nextpow2(length(config.PLSCScramLUT)-1)  CountFracLen=0  CountSampTime=1
  dataOut : Outport
  validOut : Outport  Port=2
  resetOut : Outport  Port=3
  endOfPLSC : Outport  Port=4
  wires:
  Logical Operator1/1 -> endOfPLSC/1
  Compare To Constant/1 -> Logical Operator1/1
  Data Type Conversion/1 -> Logical Operator/2
  PLSC Valid Counter/1 -> Compare To Constant/1, 1-D Lookup Table/1
  1-D Lookup Table/1 -> Data Type Conversion/1
  dataIn/1 -> Logical Operator/1
  Logical Operator/1 -> dataOut/1
  validIn/1 -> PLSC Valid Counter/2, Logical Operator1/2, validOut/1
  resetIn/1 -> PLSC Valid Counter/1, resetOut/1

== system dvbs2_stream/HDL_DUT/Tx/DVB-S2 Tx/PL Frame Generator/RAM FIFO/PL Data FIFO/Frame Length FIFO/No HDL ==
  wr : Inport
  rd : Inport  Port=2
  No HDL : Subsystem
  RAM status : MATLAB Function  TreatAsAtomicUnit=on
  wires:
  RAM status/2(ncount) -> No HDL/3(ncount)
  RAM status/1(full) -> No HDL/2(full)
  wr/1 -> No HDL/1(wr), RAM status/1(wr)
  RAM status/3(empty) -> No HDL/4(empty)
  rd/1 -> No HDL/5(rd), RAM status/2(rd)
